simulink model ""  (R2025b)
settings: Solver=ode45  StartTime=0.0  StopTime=20  RelTol=1e-3
undefined symbols (not defined in the file): DeltaT
libraries: slident x3
settings Model: Creator=USER  LastModifiedBy=francesco
settings SolverCC: AlgebraicLoopSolver=TrustRegion
settings DebuggingCC: UnconnectedInputMsg=warning  UnconnectedLineMsg=warning
settings ModelReferenceCC: EnableRefExpFcnMdlSchedulingChecks=on
settings RTWCC: GPUComputeCapability=3.5  DLArmComputeVersion=19.05

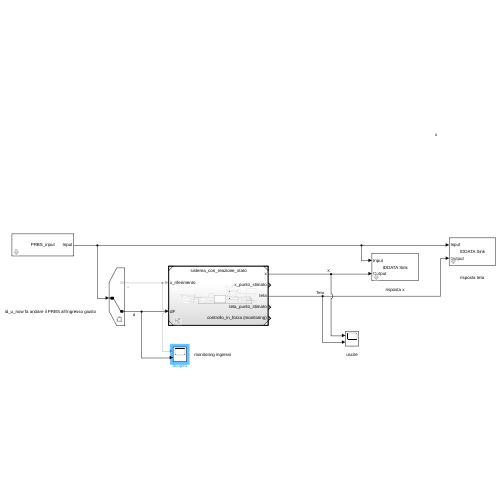
[thumbnail: Simulink's stored preview of the top-level diagram]
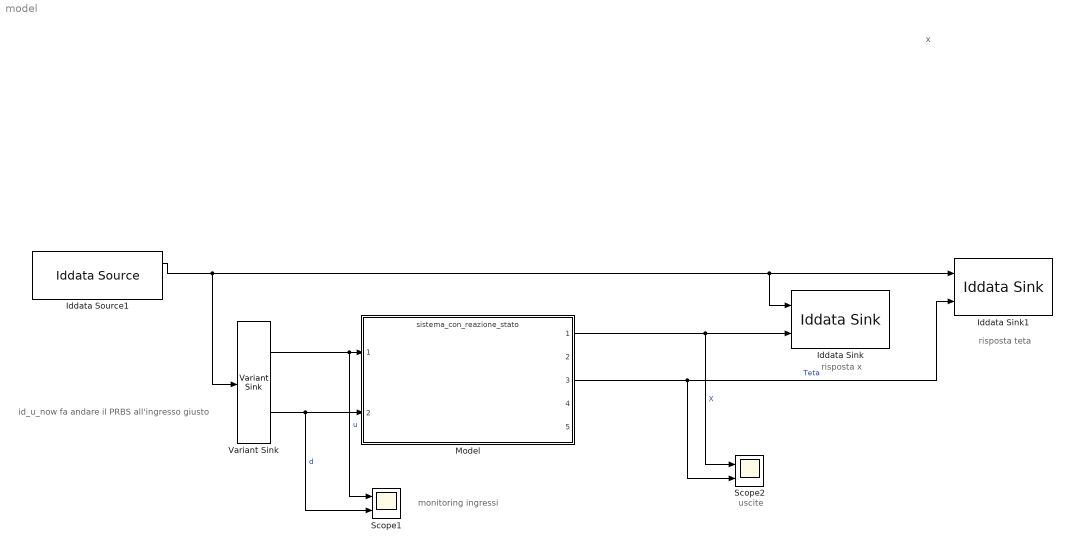
== system model ==
  note: monitoring ingressi
  note: id_u_now fa andare il PRBS all'ingresso giusto
  note: risposta teta
  note: risposta x
  note: x
  note: uscite
  Iddata Sink : slident/Iddata Sink  datasetname=IO_x  Ts=DeltaT  isu=off  isy=off
  Iddata Sink1 : slident/Iddata Sink  datasetname=IO_teta  Ts=DeltaT  isu=off  isy=off
  Iddata Source1 : slident/Iddata Source  iddataobj=PRBS_input  T0=-1
  Model : ModelReference  ModelNameDialog=sistema_con_reazione_stato.slx  SimulationMode=Normal  ModelReferenceVersion=9.55
  Scope1 : Scope  NumInputPorts=2
      settings: ActiveDisplayYMinimum=-1.25  ActiveDisplayYMaximum=1.25
  Scope2 : Scope  NumInputPorts=2
      settings: ActiveDisplayYMinimum=-0.060113003787620641  ActiveDisplayYMaximum=0.044991800627960682  DataLoggingVariableName=ScopeData2
  Variant Sink : VariantSink  VariantControls={id_u_now == 1, id_u_now == 0}
  wires:
  Model/1 -> Iddata Sink/2, Scope2/1  "X"
  Model/3 -> Iddata Sink1/2, Scope2/2  "Teta"
  Iddata Source1/1 -> Iddata Sink1/1, Iddata Sink/1, Variant Sink/1
  Variant Sink/2 -> Model/2, Scope1/2  "d"
  Variant Sink/1 -> Scope1/1, Model/1  "u"
